simulink model "LimitChecking_Average"  (R2014a)
settings: Solver=FixedStepDiscrete  StartTime=0.0  StopTime=inf  FixedStep=sample_time  RelTol=1e-3
undefined symbols (not defined in the file or in its folder): limit_gradient
libraries: visionstatistics x1, simulink x1, dspbuff3 x1
settings Model: Creator=georg  LastModifiedBy=georg

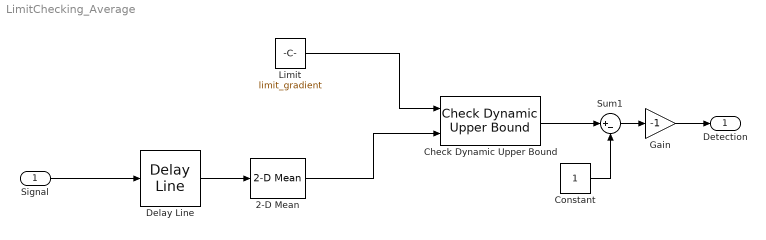
== system LimitChecking_Average ==
  Signal : Inport
  2-D Mean : visionstatistics/2-D Mean  run=off  reset_popup=None  directionMode=Entire input  dimension=1  treatSBRowAsCol=on  roiEnable=off  roiType=Rectangles  roiPortion=Entire ROI  roiOutput=Individual statistics for each ROI  roiFlag=off  outputDataTypeStr=Inherit: Same as accumulator  outputLastDataTypeStr=Inherit: Same as accumulator  outputMin=[]  outputMax=[]  accumMode=Binary point scaling  accumWordLength=32  accumFracLength=0  accumDataTypeStr=fixdt([],32,0)  accumLastDataTypeStr=fixdt([],32,0)  roundingMode=Floor  overflowMode=off
  Check Dynamic Upper Bound : simulink/Model Verification/Check Dynamic  Upper Bound  Description=sig < max  enabled=on  stopWhenAssertionFail=off  export=on  icon=graphic
  Constant : Constant
  Delay Line : dspbuff3/Delay Line  siz=20  ic=0  directfeed=on  enable_output=off  hold_output=off  TreatMby1Signals=One channel
  Gain : Gain  Gain=-1
  Limit : Constant  Value=limit_gradient
  Sum1 : Sum  Inputs=|+-
  Detection : Outport
  wires:
  Check Dynamic Upper Bound/1 -> Sum1/1
  Limit/1 -> Check Dynamic Upper Bound/1
  Constant/1 -> Sum1/2
  Sum1/1 -> Gain/1
  Gain/1 -> Detection/1
  Signal/1 -> Delay Line/1
  Delay Line/1 -> 2-D Mean/1
  2-D Mean/1 -> Check Dynamic Upper Bound/2
